simulink model "HVDCMMCInterconnection"  (R2024b)
settings: Solver=FixedStepDiscrete  StartTime=0.0  StopTime=11  RelTol=1e-3
PreLoadFcn:
  | GFLParameters_400Kv
  | HVDCMMCInterconnectionParam
StartFcn:
  | tic
StopFcn:
  | toc
values from neighbouring files (symbols this model uses):
  C_PM = 1.758e-3    (= 0.001758)    [HVDCMMCInterconnectionParam.m]
  Cfilter = 1/(Larm*wc2)    (= 4.78421193241e-05)    [HVDCMMCInterconnectionParam.m]
  Cg = 50e-9    (= 5e-08)    [HVDCMMCInterconnectionParam.m]
  Fc = Fnom*3.37    (= 168.5)    [HVDCMMCInterconnectionParam.m]
  Fnom = 50    [GFLParameters_400Kv.m]    (also in HVDCMMCInterconnectionParam.m)
  L_cable = 15e-3    (= 0.015)    [HVDCMMCInterconnectionParam.m]
  Larm = Larm_pu*(Zbase/(2*pi*Fnom))    (= 0.0529455974536)    [HVDCMMCInterconnectionParam.m]
  Limits_Qreg = [ 0.25, -0.25 ]    [HVDCMMCInterconnectionParam.m]
  Lxfo = 0.12    [HVDCMMCInterconnectionParam.m]
  Nb_PM = 36    [HVDCMMCInterconnectionParam.m]
  Pnom = 1000e6    (= 1000000000)    [HVDCMMCInterconnectionParam.m]
  Psc = Pnom*20    (= 20000000000)    [HVDCMMCInterconnectionParam.m]    (also in HVDCMMC_RunFaultAnalysis.m = gridSCLArray(k))
  R_cable = 0.5    [HVDCMMCInterconnectionParam.m]
  R_startup = 400    [HVDCMMCInterconnectionParam.m]
  Rarm = Rarm_pu*Zbase    (= 0.1663335)    [HVDCMMCInterconnectionParam.m]
  Rfilter = 1/(Cfilter*w)*30    (= 1996.002)    [HVDCMMCInterconnectionParam.m]
  Rg = 100    [HVDCMMCInterconnectionParam.m]
  Rxfo = 0.003    [HVDCMMCInterconnectionParam.m]
  Slope_Pref = 0.5    [HVDCMMCInterconnectionParam.m]
  Slope_Qref = 0.5    [HVDCMMCInterconnectionParam.m]
  Slope_Vdc_ref = Vnom_dc/5    (= 128000)    [HVDCMMCInterconnectionParam.m]
  Tbrk1_On = 0.1    [HVDCMMCInterconnectionParam.m]
  Tbrk2_On = 1.0    (= 1)    [HVDCMMCInterconnectionParam.m]
  Tdeblock = 1.5    [HVDCMMCInterconnectionParam.m]
  Tfault = 9999    [HVDCMMCInterconnectionParam.m]
  Ton_Converter2 = 4    [HVDCMMCInterconnectionParam.m]
  Ton_PQreg = 4    [HVDCMMCInterconnectionParam.m]
  Ton_VDCreg = 1.5    [HVDCMMCInterconnectionParam.m]
  Ts = Ts_Control    (= 4e-05)    [HVDCMMCInterconnectionParam.m]
  Ts_Power = 20e-6    (= 2e-05)    [HVDCMMCInterconnectionParam.m]
  Vnom_dc = 640e3    (= 640000)    [HVDCMMCInterconnectionParam.m]
  Vnom_prim = 400e3    (= 400000)    [HVDCMMCInterconnectionParam.m]
  Vnom_sec = 333e3    (= 333000)    [HVDCMMCInterconnectionParam.m]
undefined symbols (not defined in the file or in its folder): ConvCtrl, ConvPlt, DiscIntNeverNeededParam, Discrete, ee_sli_rtmsupport, Fault, gcbh, gridInverter, magnitude, Pcc, PlantSim, sps, sps_rtmsupport, spsPLL3phModel, TL, Trf
libraries: powerlib_extras x27, spsSeriesRLCBranchLib x27, simulink x14, eeGeneralControl x11, spsCurrentMeasurementLib x11, spsVoltageMeasurementLib x8, spsBreakerLib x7, eeTransforms x6, spsHalfBridgeMMCLib x6, spsSecondOrderFilterLib x4, spsabctodq0Lib x4, spsThreePhaseVIMeasurementLib x4
(part 1 of 6)
settings Model: SimulationMode=accelerator  Creator=The MathWorks, Inc.  LastModifiedBy=ke416
settings SolverCC: AlgebraicLoopSolver=TrustRegion  AutoInsertRateTranBlk=on
settings DataIOCC: SaveOutput=off  DSMLogging=off  SaveTime=off  ReturnWorkspaceOutputsName=outData
settings OptimizationCC: ReuseModelBlockBuffer=off  ExpressionDepthLimit=2147483647  LifeSpan=inf
settings DebuggingCC: CheckSSInitialOutputMsg=off  UnderspecifiedInitializationDetection=Classic  MergeDetectMultiDrivingBlocksExec=none  SolverPrmCheckMsg=warning  FcnCallInpInsideContextMsg=warning  UnconnectedInputMsg=warning  UnconnectedOutputMsg=warning  UnconnectedLineMsg=warning  AllowSymbolicDim=off  StateNameClashWarn=warning  SFUnexpectedBacktrackingDiag=warning  SFNoUnconditionalDefaultTransitionDiag=warning  SFExecutionAtInitializationDiag=none  ArithmeticOperatorsInVariantConditions=warning
settings HardwareCC: ProdBitPerPointer=32  ProdBitPerSizeT=32  ProdBitPerPtrDiffT=32  ProdLargestAtomicFloat=None  ProdIntDivRoundTo=Undefined  ProdEndianess=Unspecified  ProdWordSize=32  ProdHWDeviceType=32-bit Generic
settings ModelReferenceCC: EnableRefExpFcnMdlSchedulingChecks=on  PropagateSignalLabelsOutOfModel=off
settings SFSimCC: SimUseLocalCustomCode=off  CustomCodeUndefinedFunction=UseInterfaceOnly
settings RTWCC: RTWUseLocalCustomCode=off  GPUComputeCapability=3.5
settings CodeAppCC: StateflowObjectComments=on
settings GRTTargetCC: TargetLangStandard=C89/C90 (ANSI)  CombineOutputUpdateFcns=off  GRTInterface=on
settings ConfigComp: CovMetricSettings=dw  CovSaveCumulativeToWorkspaceVar=on  CovSaveSingleToWorkspaceVar=on  CovExternalEMLEnable=off
settings SimscapeCC: SimscapeNormalizeSystem=off

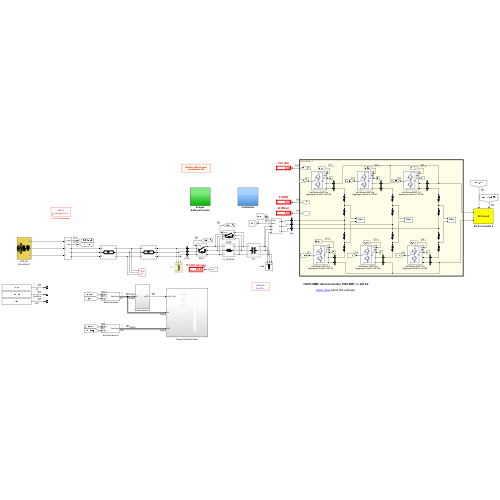
[thumbnail: Simulink's stored preview of the top-level diagram]
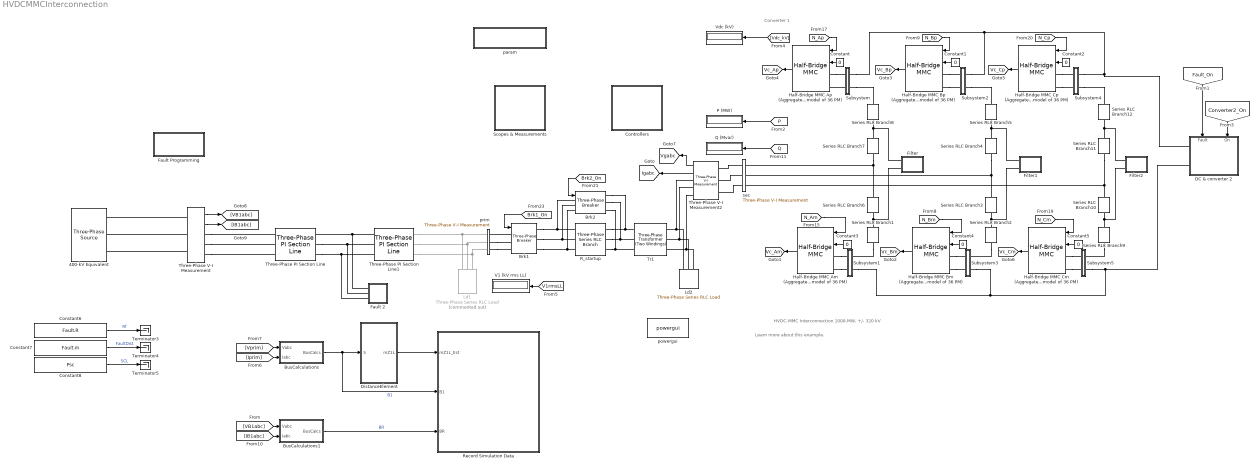
== system HVDCMMCInterconnection ==
  note: Converter 1
  note: HVDC-MMC Interconnection 1000-MW, +/- 320 kV
  note: Learn more about this example.
  400-kV Equivalent : spsThreePhaseSourceLib/Three-Phase Source  InternalConnection=Yg  VoltagePhases=off  Voltage=Vnom_prim*0.99  PhaseAngle=0  Voltage_phases=[25e3 25e3 25e3]/sqrt(3)  PhaseAngles_phases=[0 -120 +120]  Frequency=Fnom  NonIdealSource=on  SpecifyImpedance=on  Resistance=0.8929  Inductance=16.58e-3  ShortCircuitLevel=Psc  BaseVoltage=Vnom_prim  XRratio=7  BusType=swing  Pref=0  Qref=0  Prefabc=[10e3, 10e3, 10e3]  Qrefabc=[0, 0, 0]  Qmin=-inf  Qmax=inf
  Brk1 : spsThreePhaseBreakerLib/Three-Phase Breaker  InitialState=open  SwitchA=on  SwitchB=on  SwitchC=on  SwitchTimes=0.1  External=on  BreakerResistance=0.001  SnubberResistance=1e6  SnubberCapacitance=inf  Measurements=None
  Brk2 : spsThreePhaseBreakerLib/Three-Phase Breaker  InitialState=open  SwitchA=on  SwitchB=on  SwitchC=on  SwitchTimes=[30/60]*10000  External=on  BreakerResistance=0.01  SnubberResistance=1e6  SnubberCapacitance=inf  Measurements=None
  BusCalculations : Subsystem  mask{Freq=PlantSim.Freq, Ts=PlantSim.Ts}
      mask prompts: Freq "Nominal Frequency (Hz):"; Ts "Sampling Time (s):"
  BusCalculations1 : Subsystem  mask{Freq=PlantSim.Freq, Ts=PlantSim.Ts}
      mask prompts: Freq "Nominal Frequency (Hz):"; Ts "Sampling Time (s):"
  Constant{,1..5} (6 alike) : Constant  Value=0
  Constant6 : Constant  Value=Fault.R  SampleTime=-1
  Constant7 : Constant  Value=Fault.m  SampleTime=-1
  Constant8 : Constant  Value=Psc  SampleTime=-1
  Controllers : Subsystem
  DC & converter 2 : Subsystem
      settings: PortSchema="{\"entries\":[{\"content\":{\"sides\":[{\"content\":{\"connectorIds\":[\"LConn1\",\"LConn2\"]},\"type\":\"ConnectorPlacement.EquallySpacedRectSide\",\"uuid\":\"7a2c87ad-91de-4512-ad2a-35713ffc2c67\"},{\"content\":{\"connectorIds\":[],\"side\":\"RIGHT\"},\"type\":\"ConnectorPlacement.EquallySpacedRectSide\",\"uuid\":\"a4d51b8d-9b80-4f56-8990-d227af10d4d9\"},{\"content\":{\"connectorIds\":[\"In1\",\"In2\"],\"side\":\"TOP\"},\"type\":\"ConnectorPlacement.EquallySpacedRectSide\",\"uuid\":\"21e823e1-439d-404c-83ef-6279f9df48a0\"}]},\"type\":\"ConnectorPlacement.EquallySpacedConnector\",\"uuid\":\"7be36849-7bc6-4892-aa95-a5e675f45e41\"}],\"packageUris\":[\"http://schema.mathworks.com/mf0/Connector/R2020b\"],\"version\":\"1.0\"}"
      mask Display: disp('DC circuit')
  DistanceElement : Subsystem
  Fault 2 : Subsystem  mask(Fault Breaker){Ts=Ts_Power}
      mask prompts: Ts "Sample time:"
      mask Display: disp('Fault\n L1')
  Fault Programming : Subsystem  mask(Fault programming){FaultType=ABC-G, FaultLocation=L1: Protected line, ParT=[Fault.StartTime Fault.EndTime], Ts=Ts_Power}
      mask prompts: FaultType "Fault type:"; FaultLocation "Fault Location:"; ParT "Fault timing (s): [ Ton  Toff ]"; Ts "Sample time:"
      mask init:
      | switch FaultType
      | case 1
      | str='NO Fault';
      | case 2
      | str='A-G';
      | case 3
      | str='AB';
      | case 4
      | str='AB-G';
      | case 5
      | str='ABC';
      | case 6
      | str='ABC-G';
      | end
      | switch FaultLocation
      | case 1
      | str1='Protected line (L1)';
      | case 2
      | str1='Parallel line (L2)';
      | end
      | str2=sprintf('%s\n%s',str,str1);
      | Ton=ParT(1);
      | Toff=ParT(2);
      mask TypeOptions FaultType: No fault | A-G | AB | AB-G | ABC | ABC-G
      mask TypeOptions FaultLocation: L1: Protected line | L2: Parallel line
      mask Display: disp(str2)
  Filter : Subsystem
      mask Display: disp('Filter')
  Filter1 : Subsystem
      mask Display: disp('Filter')
  Filter2 : Subsystem
      mask Display: disp('Filter')
  Half-Bridge MMC Am (Aggregate model of 36 PM) : spsHalfBridgeMMCLib/Half-Bridge MMC  ModelType=Aggregate model  n=36  C=C_PM  Vc_Initial=Vc0_PM  Ron=1e-3  Rs=1e6  Cs=inf  Ron_Diode=1e-3  Rs_Diode=1e6  Cs_Diode=inf  Vf_Diode=1e-3  Rs_CurrentSource=inf  Ts=Ts_Power
  Half-Bridge MMC Ap (Aggregate model of 36 PM) : spsHalfBridgeMMCLib/Half-Bridge MMC  ModelType=Aggregate model  n=36  C=C_PM  Vc_Initial=Vc0_PM  Ron=1e-3  Rs=1e6  Cs=inf  Ron_Diode=1e-3  Rs_Diode=1e6  Cs_Diode=inf  Vf_Diode=1e-3  Rs_CurrentSource=inf  Ts=Ts_Power
  Half-Bridge MMC Bm (Aggregate model of 36 PM) : spsHalfBridgeMMCLib/Half-Bridge MMC  ModelType=Aggregate model  n=36  C=C_PM  Vc_Initial=Vc0_PM  Ron=1e-3  Rs=1e6  Cs=inf  Ron_Diode=1e-3  Rs_Diode=1e6  Cs_Diode=inf  Vf_Diode=1e-3  Rs_CurrentSource=inf  Ts=Ts_Power
  "Half-Bridge MMC Bp (Aggregate model of 36 PM) " : spsHalfBridgeMMCLib/Half-Bridge MMC  ModelType=Aggregate model  n=36  C=C_PM  Vc_Initial=Vc0_PM  Ron=1e-3  Rs=1e6  Cs=inf  Ron_Diode=1e-3  Rs_Diode=1e6  Cs_Diode=inf  Vf_Diode=1e-3  Rs_CurrentSource=inf  Ts=Ts_Power
  Half-Bridge MMC Cm (Aggregate model of 36 PM) : spsHalfBridgeMMCLib/Half-Bridge MMC  ModelType=Aggregate model  n=36  C=C_PM  Vc_Initial=Vc0_PM  Ron=1e-3  Rs=1e6  Cs=inf  Ron_Diode=1e-3  Rs_Diode=1e6  Cs_Diode=inf  Vf_Diode=1e-3  Rs_CurrentSource=inf  Ts=Ts_Power
  Half-Bridge MMC Cp (Aggregate model of 36 PM) : spsHalfBridgeMMCLib/Half-Bridge MMC  ModelType=Aggregate model  n=36  C=C_PM  Vc_Initial=Vc0_PM  Ron=1e-3  Rs=1e6  Cs=inf  Ron_Diode=1e-3  Rs_Diode=1e6  Cs_Diode=inf  Vf_Diode=1e-3  Rs_CurrentSource=inf  Ts=Ts_Power
  Ld1 : spsThreePhaseSeriesRLCLoadLib/Three-Phase Series RLC Load  Commented=on  LConnTagsString=A|B|C  Configuration=Y (grounded)  NominalVoltage=Vnom_prim  Vabc=[1e3 1e3 1e3]  Vabcp=[1e3 1e3 1e3]  NominalFrequency=Fnom  UnbalancedPower=off  ActivePower=P_Ld1  InductivePower=0  CapacitivePower=0  Pabc=[10e3 9e3 11e3]  QLabc=[100 90 110]  QCabc=[100 90 110]  Pabcp=[10e3 9e3 11e3]  QLabcp=[100 90 110]  QCabcp=[100 90 110]  Measurements=None  LoadType=constant Z
  Ld2 : spsThreePhaseSeriesRLCLoadLib/Three-Phase Series RLC Load  LConnTagsString=A|B|C  Configuration=Y (grounded)  NominalVoltage=Vnom_sec  Vabc=[1e3 1e3 1e3]  Vabcp=[1e3 1e3 1e3]  NominalFrequency=Fnom  UnbalancedPower=off  ActivePower=500e3  InductivePower=0  CapacitivePower=0  Pabc=[10e3 9e3 11e3]  QLabc=[100 90 110]  QCabc=[100 90 110]  Pabcp=[10e3 9e3 11e3]  QLabcp=[100 90 110]  QCabcp=[100 90 110]  Measurements=None  LoadType=constant Z
  P (MW) : Display
      settings: Format=bank  Decimation=5000
  Q (Mvar) : Display
      settings: Format=bank  Decimation=5000
  R_startup : spsThreePhaseSeriesRLCBranchLib/Three-Phase Series RLC Branch  LConnTagsString=A|B|C  RConnTagsString=A|B|C  BranchType=R  Resistance=R_startup  Inductance=Vnom_prim^2 / Pcc / (2*pi*Fnom)  Capacitance=1e-6  Measurements=None
  Record Simulation Data : Subsystem
  Scopes & Measurements : Subsystem
  Series RLC Branch{1..12} (12 alike) : spsSeriesRLCBranchLib/Series RLC Branch  LConnTagsString=__new0  RConnTagsString=__new0  BranchType=RL  Resistance=Rarm/2  Inductance=Larm/2  SetiL0=off  InitialCurrent=0  Capacitance=1e-6  Setx0=off  InitialVoltage=0  Measurements=None
  Subsystem : Subsystem
  Subsystem1 : Subsystem
  Subsystem2 : Subsystem
  Subsystem3 : Subsystem
  Subsystem4 : Subsystem
  Subsystem5 : Subsystem
  Terminator3 : Terminator
  Terminator4 : Terminator
  Terminator5 : Terminator
  Three-Phase PI Section Line : spsThreePhasePISectionLineLib/Three-Phase PI Section Line  LConnTagsString=a|b|c  RConnTagsString=A|B|C  Length=100*(1-Fault.m)  Frequency=Fnom  Resistances=[ 0.01273 0.3864]  Inductances="[ 0.9337e-3  4.1264e-3]"  Capacitances=[12.74e-9 7.751e-9]
  Three-Phase PI Section Line1 : spsThreePhasePISectionLineLib/Three-Phase PI Section Line  LConnTagsString=a|b|c  RConnTagsString=A|B|C  Length=100*Fault.m  Frequency=Fnom  Resistances=[ 0.01273 0.3864]  Inductances="[ 0.9337e-3  4.1264e-3]"  Capacitances=[12.74e-9 7.751e-9]
  Three-Phase V-I Measurement : spsThreePhaseVIMeasurementLib/Three-Phase V-I Measurement  VoltageMeasurement=phase-to-ground  SetLabelV=off  LabelV=Vabc  Vpu=off  VpuLL=off  CurrentMeasurement=yes  SetLabelI=off  LabelI=Iabc  Ipu=off  Pbase=100e6  Vbase=500e3  OutputType=Complex  PhasorSimulation=off  PSBequivalent=0
  Three-Phase V-I Measurement2 : spsThreePhaseVIMeasurementLib/Three-Phase V-I Measurement  VoltageMeasurement=phase-to-ground  SetLabelV=off  LabelV=Vabc  Vpu=off  VpuLL=off  CurrentMeasurement=yes  SetLabelI=off  LabelI=Iabc  Ipu=off  Pbase=100e6  Vbase=500e3  OutputType=Complex  PhasorSimulation=off  PSBequivalent=0
  Tr1 : spsThreePhaseTransformerTwoWindingsLib/Three-Phase Transformer (Two Windings)  Winding1Connection=Yg  Winding2Connection=Y  CoreType=Three single-phase transformers  SetSaturation=off  Hysteresis=off  DataFile='hysteresis'  SetInitialFlux=off  Measurements=None  UNITS=pu  NominalPower=[ Pnom , Fnom ]  Winding1="[ Vnom_prim , Rxfo/2,  Lxfo/2 ]"  Winding2="[ Vnom_sec , Rxfo/2,  Lxfo/2 ]"  Rm=1000  Lm=1000  L0=0.5  Saturation=[ 0,0 ; 0.0024,1.2 ; 1.0,1.52 ]  InitialFluxes=[ 0.8 , -0.8 , 0.7 ]  BreakLoop=off  DiscreteSolver=Trapezoidal iterative  DataType=off  TransfoNumber=1
  V1 (kV rms LL) : Display
      settings: Format=bank  Decimation=5000
  Vdc (kV) : Display
      settings: Format=bank  Decimation=5000
  param : Subsystem
      settings: OpenFcn=open('HVDCMMCInterconnectionParam')
      mask Display: disp('Double-click to open\nparameters file')
  powergui : spspowerguiLib/powergui  Priority=1  SimulationMode=Discrete  SampleTime=Ts_Power  frequency=60  Iterations=50  frequencyindice=0  Pbase=100e6  ErrMax=1e-4  UnitsV=kV  UnitsW=MW  buscounter=0  FunctionMessages=off  echomessages=off  EnableUseOfTLC=off  CurrentSourceSwitches=off  DisableSnubberDevices=off  DisableRonSwitches=off  DisableVfSwitches=off  DisplayEquations=off  AutomaticDiscreteSolvers=off  SolverType=Tustin/Backward Euler (TBE)  Interpol=off  ExternalGateDelay=off  methode=off  Ts=10  x0status=blocks  SPID=off  SwTol=0  HookPort=off  NonlinearTolerance=1e-4  nMaxIteration=100  ContinueOnMaxIteration=off  RestoreLinks=warning  ResistiveCurrentMeasurement=off  Frange=[0:2:500]  Ylog=off  Xlog=on  ShowGrid=off  save=off  variable=ZData  structure=VIprim  ZoomFFT=on  StartTime=0.15  cycles=2  DisplayStyle=1  fundamental=50  FreqAxis=on  MaxFrequency=1000  frequencyindicesteady=1  RmsSteady=1  display=off
  prim : spsThreePhaseVIMeasurementLib/Three-Phase V-I Measurement  VoltageMeasurement=phase-to-ground  SetLabelV=on  LabelV=Vprim  Vpu=off  VpuLL=off  CurrentMeasurement=yes  SetLabelI=on  LabelI=Iprim  Ipu=off  Pbase=100e6  Vbase=500e3  OutputType=Complex  PhasorSimulation=off  PSBequivalent=0
  sec : spsThreePhaseVIMeasurementLib/Three-Phase V-I Measurement  VoltageMeasurement=phase-to-ground  SetLabelV=on  LabelV=Vsec  Vpu=off  VpuLL=off  CurrentMeasurement=yes  SetLabelI=on  LabelI=Isec  Ipu=off  Pbase=100e6  Vbase=500e3  OutputType=Complex  PhasorSimulation=off  PSBequivalent=0
  tag scope: Igabc=global, Vc_Am=global, Vc_Ap=global, Vc_Bm=global, Vc_Bp=global, Vc_Cm=global, Vc_Cp=global, Vgabc=global
  wires:
  [P] -> P (MW)/1
  [N_Cp] -> Half-Bridge MMC Cp (Aggregate model of 36 PM)/1
  Half-Bridge MMC Cp (Aggregate model of 36 PM)/1 -> [Vc_Cp]
  Half-Bridge MMC Am (Aggregate model of 36 PM)/1 -> [Vc_Am]
  Half-Bridge MMC Bm (Aggregate model of 36 PM)/1 -> [Vc_Bm]
  Half-Bridge MMC Cm (Aggregate model of 36 PM)/1 -> [Vc_Cm]
  [N_Bm] -> Half-Bridge MMC Bm (Aggregate model of 36 PM)/1
  [Brk2_On] -> Brk2/1
  [Vdc_kV] -> Vdc (kV)/1
  [V1rmsLL] -> V1 (kV rms LL)/1
  [Q] -> Q (Mvar)/1
  Half-Bridge MMC Ap (Aggregate model of 36 PM)/1 -> [Vc_Ap]
  [Converter2_On] -> DC & converter 2/2(On)
  [Fault_On] -> DC & converter 2/1(Fault)
  [N_Ap] -> Half-Bridge MMC Ap (Aggregate model of 36 PM)/1
  [N_Am] -> Half-Bridge MMC Am (Aggregate model of 36 PM)/1
  "Half-Bridge MMC Bp (Aggregate model of 36 PM) "/1 -> [Vc_Bp]
  [N_Bp] -> "Half-Bridge MMC Bp (Aggregate model of 36 PM) "/1
  [N_Cm] -> Half-Bridge MMC Cm (Aggregate model of 36 PM)/1
  Constant/1 -> Half-Bridge MMC Ap (Aggregate model of 36 PM)/2
  Constant1/1 -> "Half-Bridge MMC Bp (Aggregate model of 36 PM) "/2
  Constant2/1 -> Half-Bridge MMC Cp (Aggregate model of 36 PM)/2
  Constant3/1 -> Half-Bridge MMC Am (Aggregate model of 36 PM)/2
  Constant4/1 -> Half-Bridge MMC Bm (Aggregate model of 36 PM)/2
  Constant5/1 -> Half-Bridge MMC Cm (Aggregate model of 36 PM)/2
  Three-Phase V-I Measurement2/1 -> [Vgabc]
  Three-Phase V-I Measurement2/2 -> [Igabc]
  [Brk1_On] -> Brk1/1
  BusCalculations/1(BusCalcs) -> Record Simulation Data/2(B1), DistanceElement/1(S)  "B1"
  Constant8/1 -> Terminator5/1  "SCL"
  DistanceElement/1(mZ1L) -> Record Simulation Data/1(mZ1L_Est)
  Constant7/1 -> Terminator4/1  "FaultDist"
  Constant6/1 -> Terminator3/1  "Rf"
  [Iprim] -> BusCalculations/2(Iabc)
  [Vprim] -> BusCalculations/1(Vabc)
  BusCalculations1/1(BusCalcs) -> Record Simulation Data/3(BR)  "BR"
  [VB1abc] -> BusCalculations1/1(Vabc)
  [IB1abc] -> BusCalculations1/2(Iabc)
  Three-Phase V-I Measurement/2 -> [IB1abc]
  Three-Phase V-I Measurement/1 -> [VB1abc]
  connections:
  Ld1/LConn1 -- Three-Phase PI Section Line1/RConn1 -- prim/RConn1
  Ld1/LConn2 -- Three-Phase PI Section Line1/RConn2 -- prim/RConn2
  Ld1/LConn3 -- Three-Phase PI Section Line1/RConn3 -- prim/RConn3
  Series RLC Branch7/RConn1 -- Series RLC Branch6/LConn1 -- sec/LConn1
  Series RLC Branch1/LConn1 -- Filter/LConn2 -- Series RLC Branch6/RConn1
  Series RLC Branch7/LConn1 -- Filter/LConn1 -- Series RLC Branch8/RConn1
  Half-Bridge MMC Ap (Aggregate model of 36 PM)/LConn1 -- Subsystem/LConn1
  Subsystem/LConn2 -- Half-Bridge MMC Ap (Aggregate model of 36 PM)/LConn2
  Subsystem/RConn2 -- Series RLC Branch8/LConn1
  Half-Bridge MMC Am (Aggregate model of 36 PM)/LConn2 -- Subsystem1/LConn2
  Half-Bridge MMC Am (Aggregate model of 36 PM)/LConn1 -- Subsystem1/LConn1
  Series RLC Branch1/RConn1 -- Subsystem1/RConn1
  Series RLC Branch4/RConn1 -- Series RLC Branch3/LConn1 -- sec/LConn2
  Filter1/LConn2 -- Series RLC Branch2/LConn1 -- Series RLC Branch3/RConn1
  Series RLC Branch4/LConn1 -- Filter1/LConn1 -- Series RLC Branch5/RConn1
  "Half-Bridge MMC Bp (Aggregate model of 36 PM) "/LConn2 -- Subsystem2/LConn2
  "Half-Bridge MMC Bp (Aggregate model of 36 PM) "/LConn1 -- Subsystem2/LConn1
  Subsystem2/RConn2 -- Series RLC Branch5/LConn1
  Series RLC Branch2/RConn1 -- Subsystem3/RConn1
  Half-Bridge MMC Bm (Aggregate model of 36 PM)/LConn1 -- Subsystem3/LConn1
  Half-Bridge MMC Bm (Aggregate model of 36 PM)/LConn2 -- Subsystem3/LConn2
  Series RLC Branch11/RConn1 -- Series RLC Branch10/LConn1 -- sec/LConn3
  Series RLC Branch10/RConn1 -- Filter2/LConn2 -- Series RLC Branch9/LConn1
  Series RLC Branch12/RConn1 -- Series RLC Branch11/LConn1 -- Filter2/LConn1
  Half-Bridge MMC Cp (Aggregate model of 36 PM)/LConn1 -- Subsystem4/LConn1
  Half-Bridge MMC Cm (Aggregate model of 36 PM)/LConn1 -- Subsystem5/LConn1
  Half-Bridge MMC Cm (Aggregate model of 36 PM)/LConn2 -- Subsystem5/LConn2
  Subsystem4/RConn2 -- Series RLC Branch12/LConn1
  Half-Bridge MMC Cp (Aggregate model of 36 PM)/LConn2 -- Subsystem4/LConn2
  Series RLC Branch9/RConn1 -- Subsystem5/RConn1
  Subsystem/RConn1 -- Subsystem4/RConn1 -- DC & converter 2/LConn1 -- Subsystem2/RConn1
  Subsystem1/RConn2 -- Subsystem5/RConn2 -- DC & converter 2/LConn2 -- Subsystem3/RConn2
  Ld2/LConn1 -- Three-Phase V-I Measurement2/RConn1 -- Tr1/RConn1
  Ld2/LConn2 -- Three-Phase V-I Measurement2/RConn2 -- Tr1/RConn2
  Ld2/LConn3 -- Three-Phase V-I Measurement2/RConn3 -- Tr1/RConn3
  Brk2/LConn1 -- Brk1/RConn1 -- R_startup/LConn1
  Brk2/LConn2 -- Brk1/RConn2 -- R_startup/LConn2
  Brk2/LConn3 -- Brk1/RConn3 -- R_startup/LConn3
  R_startup/RConn1 -- Brk2/RConn1 -- Tr1/LConn1
  R_startup/RConn2 -- Brk2/RConn2 -- Tr1/LConn2
  R_startup/RConn3 -- Brk2/RConn3 -- Tr1/LConn3
  Three-Phase V-I Measurement/RConn2 -- Three-Phase PI Section Line/LConn2
  Three-Phase V-I Measurement/RConn1 -- Three-Phase PI Section Line/LConn1
  Three-Phase V-I Measurement/RConn3 -- Three-Phase PI Section Line/LConn3
  Three-Phase V-I Measurement/LConn3 -- 400-kV Equivalent/RConn3
  Three-Phase V-I Measurement/LConn2 -- 400-kV Equivalent/RConn2
  Three-Phase V-I Measurement/LConn1 -- 400-kV Equivalent/RConn1
  sec/RConn1 -- Three-Phase V-I Measurement2/LConn1
  sec/RConn2 -- Three-Phase V-I Measurement2/LConn2
  sec/RConn3 -- Three-Phase V-I Measurement2/LConn3
  Brk1/LConn1 -- prim/LConn1
  prim/LConn2 -- Brk1/LConn2
  prim/LConn3 -- Brk1/LConn3
  Three-Phase PI Section Line1/LConn1 -- Fault 2/LConn1 -- Three-Phase PI Section Line/RConn1
  Three-Phase PI Section Line/RConn2 -- Fault 2/LConn2 -- Three-Phase PI Section Line1/LConn2
  Three-Phase PI Section Line/RConn3 -- Fault 2/LConn3 -- Three-Phase PI Section Line1/LConn3

== system HVDCMMCInterconnection/BusCalculations ==
  Vabc : Inport
  Iabc : Inport  Port=2
  Bus Creator : BusCreator  Inputs=6
  Bus Creator3 : BusCreator  Inputs=4
  Bus Creator4 : BusCreator  Inputs=4
  Complex2Phasor : Subsystem
  Complex2Phasor1 : Subsystem
  Demux : Demux  Outputs=3
  Demux1 : Demux  Outputs=3
  Measurement Unit (Phasor Computation) : Subsystem  mask(Measurement Unit){Ts=Ts}
      mask prompts: Ts "Sample time:"
  "Power (3ph, Instantaneous)1" : spsPower3phInstantaneousLib/Power (3ph, Instantaneous)
  SymmetricalComponentsCalc : Subsystem
  SymmetricalComponentsCalc1 : Subsystem
  BusCalcs : Outport
  wires:
  Vabc/1 -> Demux/1, Measurement Unit (Phasor Computation)/1(Vabc(t)), "Power (3ph, Instantaneous)1"/1
  Iabc/1 -> Demux1/1, Measurement Unit (Phasor Computation)/2(Iabc(t)), "Power (3ph, Instantaneous)1"/2
  "Power (3ph, Instantaneous)1"/2 -> Bus Creator/6  "Q"
  Measurement Unit (Phasor Computation)/2(" Iabc_Fund") -> SymmetricalComponentsCalc1/1(abc), Complex2Phasor1/1(complex)
  Demux1/1 -> Bus Creator4/1  "a"
  Bus Creator3/1 -> Bus Creator/1  "V"
  Demux/2 -> Bus Creator3/2  "b"
  Demux1/3 -> Bus Creator4/3  "c"
  Measurement Unit (Phasor Computation)/1(Vabc_Fund) -> Complex2Phasor/1(complex), SymmetricalComponentsCalc/1(abc)
  SymmetricalComponentsCalc1/1(ABC+-0) -> Bus Creator/4  "ISymm"
  Demux/1 -> Bus Creator3/1  "a"
  SymmetricalComponentsCalc/1(ABC+-0) -> Bus Creator/2  "VSymm"
  Bus Creator4/1 -> Bus Creator/3  "I"
  Demux1/2 -> Bus Creator4/2  "b"
  "Power (3ph, Instantaneous)1"/1 -> Bus Creator/5  "P"
  Demux/3 -> Bus Creator3/3  "c"
  Bus Creator/1 -> BusCalcs/1
  Complex2Phasor/1(Phasor) -> Bus Creator3/4  "Phasor"
  Complex2Phasor1/1(Phasor) -> Bus Creator4/4  "Phasor"

== system HVDCMMCInterconnection/BusCalculations1 ==
  Vabc : Inport
  Iabc : Inport  Port=2
  Bus Creator : BusCreator  Inputs=6
  Bus Creator3 : BusCreator  Inputs=4
  Bus Creator4 : BusCreator  Inputs=4
  Complex2Phasor : Subsystem
  Complex2Phasor1 : Subsystem
  Demux : Demux  Outputs=3
  Demux1 : Demux  Outputs=3
  Measurement Unit (Phasor Computation) : Subsystem  mask(Measurement Unit){Ts=Ts}
      mask prompts: Ts "Sample time:"
  "Power (3ph, Instantaneous)1" : spsPower3phInstantaneousLib/Power (3ph, Instantaneous)
  SymmetricalComponentsCalc : Subsystem
  SymmetricalComponentsCalc1 : Subsystem
  BusCalcs : Outport
  wires:
  Complex2Phasor1/1(Phasor) -> Bus Creator4/4  "Phasor"
  Complex2Phasor/1(Phasor) -> Bus Creator3/4  "Phasor"
  Bus Creator/1 -> BusCalcs/1
  Demux/3 -> Bus Creator3/3  "c"
  "Power (3ph, Instantaneous)1"/1 -> Bus Creator/5  "P"
  Demux1/2 -> Bus Creator4/2  "b"
  Bus Creator4/1 -> Bus Creator/3  "I"
  SymmetricalComponentsCalc/1(ABC+-0) -> Bus Creator/2  "VSymm"
  Demux/1 -> Bus Creator3/1  "a"
  SymmetricalComponentsCalc1/1(ABC+-0) -> Bus Creator/4  "ISymm"
  Measurement Unit (Phasor Computation)/1(Vabc_Fund) -> SymmetricalComponentsCalc/1(abc), Complex2Phasor/1(complex)
  Demux1/3 -> Bus Creator4/3  "c"
  Demux/2 -> Bus Creator3/2  "b"
  Bus Creator3/1 -> Bus Creator/1  "V"
  Demux1/1 -> Bus Creator4/1  "a"
  Measurement Unit (Phasor Computation)/2(" Iabc_Fund") -> Complex2Phasor1/1(complex), SymmetricalComponentsCalc1/1(abc)
  "Power (3ph, Instantaneous)1"/2 -> Bus Creator/6  "Q"
  Iabc/1 -> "Power (3ph, Instantaneous)1"/2, Measurement Unit (Phasor Computation)/2(Iabc(t)), Demux1/1
  Vabc/1 -> "Power (3ph, Instantaneous)1"/1, Measurement Unit (Phasor Computation)/1(Vabc(t)), Demux/1

== system HVDCMMCInterconnection/Controllers ==
  note: HVDC-MMC Control System
  Controllers : Subsystem  Variant=on  VariantControl=Controllers
  PWM Generators & Calculation of number of inserted modules (Nin) and number of blocked module (Nbl) : Subsystem
  Rate Transition11 : RateTransition  OutPortSampleTime=Ts_Power
  Sequencer : Subsystem
      mask Display: disp('Sequencer')
  Terminator : Terminator
  Terminator1 : Terminator
  Terminator2 : Terminator
  Unit Delay{,1..5} (6 alike) : UnitDelay  SampleTime=-1  HasFrameUpgradeWarning=on
  tag scope: N_Am=global, N_Ap=global, N_Bm=global, N_Bp=global, N_Cm=global, N_Cp=global
  wires:
  Rate Transition11/1 -> PWM Generators & Calculation of number of inserted modules (Nin) and number of blocked module (Nbl)/1(Uref_ABC)
  PWM Generators & Calculation of number of inserted modules (Nin) and number of blocked module (Nbl)/1(N_Ap) -> Unit Delay/1
  PWM Generators & Calculation of number of inserted modules (Nin) and number of blocked module (Nbl)/2(N_Bp) -> Unit Delay1/1
  PWM Generators & Calculation of number of inserted modules (Nin) and number of blocked module (Nbl)/3(N_Cp) -> Unit Delay2/1
  PWM Generators & Calculation of number of inserted modules (Nin) and number of blocked module (Nbl)/4(N_Am) -> Unit Delay3/1
  PWM Generators & Calculation of number of inserted modules (Nin) and number of blocked module (Nbl)/5(N_Bm) -> Unit Delay4/1
  PWM Generators & Calculation of number of inserted modules (Nin) and number of blocked module (Nbl)/6(N_Cm) -> Unit Delay5/1
  [Blk] -> PWM Generators & Calculation of number of inserted modules (Nin) and number of blocked module (Nbl)/2(Block)
  Unit Delay/1 -> [N_Ap]
  Unit Delay1/1 -> [N_Bp]
  Unit Delay2/1 -> [N_Cp]
  Unit Delay3/1 -> [N_Am]
  Unit Delay4/1 -> [N_Bm]
  Unit Delay5/1 -> [N_Cm]
  [Pref] -> Controllers/1(PrefPU)  "Pref"
  [Qref] -> Controllers/2(QrefPU)  "Qref"
  [Vdc1] -> Controllers/3(Vdc)
  [Vgabc] -> Controllers/4(Vsec)
  [Igabc] -> Controllers/5(Isec)
  [Vprim] -> Controllers/6(VPcc)
  Controllers/1(Uref) -> Rate Transition11/1  "Uref_GFL"
  Controllers/2(Pmeas) -> Terminator/1
  Controllers/3(Qmeas) -> Terminator1/1
  Controllers/4(fmeas) -> Terminator2/1

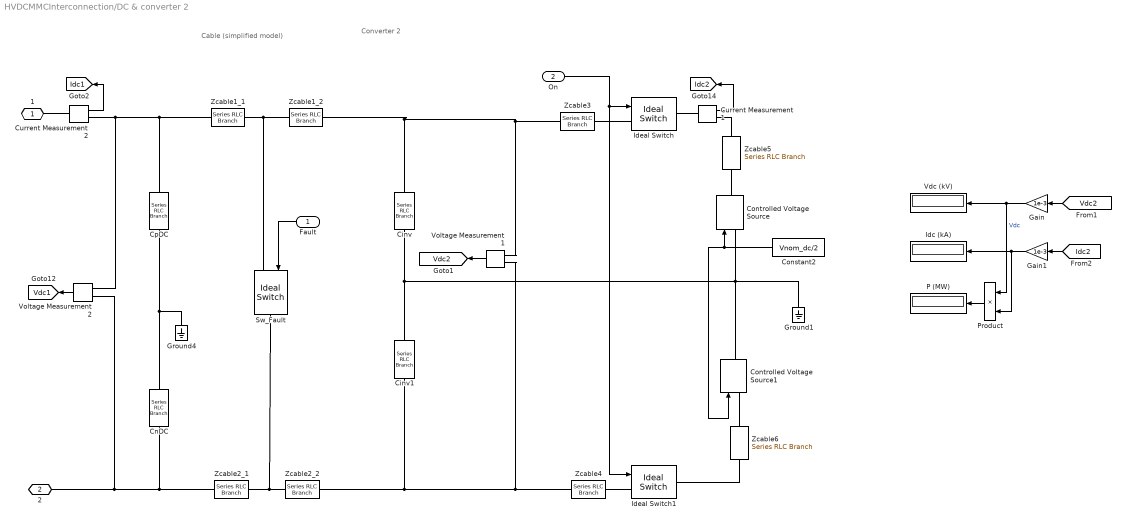
== system HVDCMMCInterconnection/DC & converter 2 ==
  note: Cable (simplified model)
  note: Converter 2
  Fault : Inport
  On : Inport  Port=2
  Cinv : spsSeriesRLCBranchLib/Series RLC Branch  LConnTagsString=__new0  RConnTagsString=__new0  BranchType=RC  Resistance=1e-3  Inductance=1e-3  SetiL0=off  InitialCurrent=0  Capacitance=C_PM/Nb_PM*3  Setx0=off  InitialVoltage=Vnom_dc/2  Measurements=None
  Cinv1 : spsSeriesRLCBranchLib/Series RLC Branch  LConnTagsString=__new0  RConnTagsString=__new0  BranchType=RC  Resistance=1e-3  Inductance=1e-3  SetiL0=off  InitialCurrent=0  Capacitance=C_PM/Nb_PM*3  Setx0=off  InitialVoltage=Vnom_dc/2  Measurements=None
  CnDC : spsSeriesRLCBranchLib/Series RLC Branch  LConnTagsString=__new0  RConnTagsString=__new0  BranchType=RC  Resistance=Rg  Inductance=1e-3  SetiL0=off  InitialCurrent=0  Capacitance=Cg  Setx0=off  InitialVoltage=Vnom_dc/2  Measurements=None
  Constant2 : Constant  Value=Vnom_dc/2  SampleTime=Ts_Power
  Controlled Voltage Source : spsControlledVoltageSourceLib/Controlled Voltage Source  Initialize=off  Source_Type=AC  Amplitude=0  Phase=0  Frequency=0  Measurements=None
  Controlled Voltage Source1 : spsControlledVoltageSourceLib/Controlled Voltage Source  Initialize=off  Source_Type=AC  Amplitude=0  Phase=0  Frequency=0  Measurements=None
  CpDC : spsSeriesRLCBranchLib/Series RLC Branch  LConnTagsString=__new0  RConnTagsString=__new0  BranchType=RC  Resistance=Rg  Inductance=1e-3  SetiL0=off  InitialCurrent=0  Capacitance=Cg  Setx0=off  InitialVoltage=Vnom_dc/2  Measurements=None
  Current Measurement1 : spsCurrentMeasurementLib/Current Measurement  PhasorSimulation=off  OutputType=Complex  PSBequivalent=0
  Current Measurement2 : spsCurrentMeasurementLib/Current Measurement  PhasorSimulation=off  OutputType=Complex  PSBequivalent=0
  Gain : Gain  Gain=1e-3
  Gain1 : Gain  Gain=1e-3
  Ground1 : spsGroundLib/Ground  LConnTagsString=a
  Ground4 : spsGroundLib/Ground  LConnTagsString=a
  Idc (kA) : Display
      settings: Format=bank  Decimation=5000
  Ideal Switch : spsIdealSwitchLib/Ideal Switch  Ron=0.001  Lon=0  IC=0  Rs=1e6  Cs=inf  Measurements=off
  Ideal Switch1 : spsIdealSwitchLib/Ideal Switch  Ron=0.001  Lon=0  IC=0  Rs=1e6  Cs=inf  Measurements=off
  P (MW) : Display
      settings: Format=bank  Decimation=5000
  Product : Product
  Sw_Fault : spsIdealSwitchLib/Ideal Switch  Ron=Rfault  Lon=0  IC=0  Rs=1e6  Cs=inf  Measurements=off
  Vdc (kV) : Display
      settings: Format=bank  Decimation=5000
  Voltage Measurement1 : spsVoltageMeasurementLib/Voltage Measurement  PhasorSimulation=off  OutputType=Complex  PSBequivalent=0
  Voltage Measurement2 : spsVoltageMeasurementLib/Voltage Measurement  PhasorSimulation=off  OutputType=Complex  PSBequivalent=0
  Zcable1_1 : spsSeriesRLCBranchLib/Series RLC Branch  LConnTagsString=__new0  RConnTagsString=__new0  BranchType=RL  Resistance=R_cable/2  Inductance=L_cable/2  SetiL0=off  InitialCurrent=0  Capacitance=1e-6  Setx0=off  InitialVoltage=0  Measurements=None
  Zcable1_2 : spsSeriesRLCBranchLib/Series RLC Branch  LConnTagsString=__new0  RConnTagsString=__new0  BranchType=RL  Resistance=R_cable/2  Inductance=L_cable/2  SetiL0=off  InitialCurrent=0  Capacitance=1e-6  Setx0=off  InitialVoltage=0  Measurements=None
  Zcable2_1 : spsSeriesRLCBranchLib/Series RLC Branch  LConnTagsString=__new0  RConnTagsString=__new0  BranchType=RL  Resistance=R_cable/2  Inductance=L_cable/2  SetiL0=off  InitialCurrent=0  Capacitance=1e-6  Setx0=off  InitialVoltage=0  Measurements=None
  Zcable2_2 : spsSeriesRLCBranchLib/Series RLC Branch  LConnTagsString=__new0  RConnTagsString=__new0  BranchType=RL  Resistance=R_cable/2  Inductance=L_cable/2  SetiL0=off  InitialCurrent=0  Capacitance=1e-6  Setx0=off  InitialVoltage=0  Measurements=None
  Zcable3 : spsSeriesRLCBranchLib/Series RLC Branch  LConnTagsString=__new0  RConnTagsString=__new0  BranchType=R  Resistance=1e-3  Inductance=1e-3  SetiL0=off  InitialCurrent=0  Capacitance=1e-6  Setx0=off  InitialVoltage=0  Measurements=None
  Zcable4 : spsSeriesRLCBranchLib/Series RLC Branch  LConnTagsString=__new0  RConnTagsString=__new0  BranchType=R  Resistance=1e-3  Inductance=1e-3  SetiL0=off  InitialCurrent=0  Capacitance=1e-6  Setx0=off  InitialVoltage=0  Measurements=None
  Zcable5 : spsSeriesRLCBranchLib/Series RLC Branch  LConnTagsString=__new0  RConnTagsString=__new0  BranchType=RL  Resistance=1e-2  Inductance=1e-4  SetiL0=off  InitialCurrent=0  Capacitance=1e-6  Setx0=off  InitialVoltage=0  Measurements=None
  Zcable6 : spsSeriesRLCBranchLib/Series RLC Branch  LConnTagsString=__new0  RConnTagsString=__new0  BranchType=RL  Resistance=1e-2  Inductance=1e-4  SetiL0=off  InitialCurrent=0  Capacitance=1e-6  Setx0=off  InitialVoltage=0  Measurements=None
  1 : PMIOPort  Side=Left
  2 : PMIOPort  Port=2  Side=Left
  tag scope: Idc1=global, Idc2=global, Vdc1=global, Vdc2=global
  wires:
  Voltage Measurement2/1 -> [Vdc1]
  Constant2/1 -> Controlled Voltage Source1/1, Controlled Voltage Source/1
  Voltage Measurement1/1 -> [Vdc2]
  Gain/1 -> Product/1, Vdc (kV)/1  "Vdc"
  Gain1/1 -> Product/2, Idc (kA)/1
  [Vdc2] -> Gain/1
  [Idc2] -> Gain1/1
  Product/1 -> P (MW)/1
  Current Measurement1/1 -> [Idc2]
  Current Measurement2/1 -> [Idc1]
  On/1 -> Ideal Switch1/1, Ideal Switch/1
  Fault/1 -> Sw_Fault/1
  connections:
  Voltage Measurement1/LConn1 -- Zcable1_2/LConn1 -- Cinv/LConn1 -- Zcable3/RConn1
  Controlled Voltage Source1/RConn1 -- Ground1/LConn1 -- Cinv1/LConn1 -- Cinv/RConn1 -- Controlled Voltage Source/LConn1
  Ground4/LConn1 -- CnDC/LConn1 -- CpDC/RConn1
  Zcable2_1/RConn1 -- CnDC/RConn1 -- Voltage Measurement2/LConn2 -- 2/RConn1
  Zcable2_2/RConn1 -- Sw_Fault/RConn1 -- Zcable2_1/LConn1
  Ideal Switch/LConn1 -- Zcable3/LConn1
  Ideal Switch1/LConn1 -- Zcable4/LConn1
  Zcable1_1/RConn1 -- Voltage Measurement2/LConn1 -- Current Measurement2/RConn1 -- CpDC/LConn1
  Ideal Switch/RConn1 -- Current Measurement1/LConn1
  Zcable5/LConn1 -- Current Measurement1/RConn1
  Zcable5/RConn1 -- Controlled Voltage Source/RConn1
  Zcable6/LConn1 -- Controlled Voltage Source1/LConn1
  Zcable6/RConn1 -- Ideal Switch1/RConn1
  1/RConn1 -- Current Measurement2/LConn1
  Zcable1_1/LConn1 -- Zcable1_2/RConn1 -- Sw_Fault/LConn1
  Zcable2_2/LConn1 -- Cinv1/RConn1 -- Zcable4/RConn1 -- Voltage Measurement1/LConn2

== system HVDCMMCInterconnection/DistanceElement ==
  S : Inport
  Abs : Abs  SaturateOnIntegerOverflow=off
  Add : Sum
  Bus Selector : BusSelector  OutputSignals=V.Phasor.a.mag,V.Phasor.a.phase,I.Phasor.a.mag,I.Phasor.a.phase,ISymm.A.mag.zero,ISymm.A.phase.zero
  Constant : Constant  Value=1+eps*1i  SampleTime=-1
  Divide : Product  Inputs=*/
  Gain : Gain  Gain=TL.K0
  Gain2 : Gain  Gain=pi/180
  Gain3 : Gain  Gain=pi/180
  Gain4 : Gain  Gain=pi/180
  Magnitude-Angle to Complex : MagnitudeAngleToComplex
  Magnitude-Angle to Complex1 : MagnitudeAngleToComplex
  Magnitude-Angle to Complex2 : MagnitudeAngleToComplex
  Switch : Switch  Criteria=u2 ~= 0  SaturateOnIntegerOverflow=off  InputSameDT=off
  mZ1L : Outport
  wires:
  Magnitude-Angle to Complex1/1 -> Add/1  "IaS"
  Bus Selector/1 -> Magnitude-Angle to Complex/1  "<mag>"
  Divide/1 -> mZ1L/1  "mZ1L_Est"
  Add/1 -> Abs/1, Switch/1  "IaS+I0SK0"
  Bus Selector/3 -> Magnitude-Angle to Complex1/1  "<mag>"
  Bus Selector/2 -> Gain2/1  "<phase>"
  Magnitude-Angle to Complex2/1 -> Gain/1  "I0S"
  Magnitude-Angle to Complex/1 -> Divide/1  "VaS"
  Gain/1 -> Add/2
  Bus Selector/4 -> Gain3/1  "<phase>"
  Bus Selector/6 -> Gain4/1  "<zero>"
  Bus Selector/5 -> Magnitude-Angle to Complex2/1  "<zero>"
  S/1 -> Bus Selector/1
  Gain2/1 -> Magnitude-Angle to Complex/2
  Gain3/1 -> Magnitude-Angle to Complex1/2
  Gain4/1 -> Magnitude-Angle to Complex2/2
  Constant/1 -> Switch/3
  Switch/1 -> Divide/2
  Abs/1 -> Switch/2

== system HVDCMMCInterconnection/Fault 2 ==
  BreakerA : spsBreakerLib/Breaker  InitialState=0  SwitchingTimes="[ 4/60  5/60 ]"  External=on  BreakerResistance=0.001  SnubberResistance=1e6  SnubberCapacitance=inf  Measurements=None  MoreParameters=off  NoBreakLoop=off
      settings: AttributesFormatString=\n
  BreakerB : spsBreakerLib/Breaker  InitialState=0  SwitchingTimes="[ 4/60  5/60 ]"  External=on  BreakerResistance=0.001  SnubberResistance=1e6  SnubberCapacitance=inf  Measurements=None  MoreParameters=off  NoBreakLoop=off
      settings: AttributesFormatString=\n
  BreakerC : spsBreakerLib/Breaker  InitialState=0  SwitchingTimes="[ 4/60  5/60 ]"  External=on  BreakerResistance=0.001  SnubberResistance=1e6  SnubberCapacitance=inf  Measurements=None  MoreParameters=off  NoBreakLoop=off
      settings: AttributesFormatString=\n
  BreakerN : spsBreakerLib/Breaker  InitialState=0  SwitchingTimes="[ 4/60  5/60 ]"  External=on  BreakerResistance=0.001  SnubberResistance=1e6  SnubberCapacitance=inf  Measurements=None  MoreParameters=off  NoBreakLoop=off
      settings: AttributesFormatString=\n
  Demux : Demux
      settings: DisplayOption=none
  Ground : spsGroundLib/Ground  LConnTagsString=a  RConnTagsString=__newr0
  Series RLC Branch : spsSeriesRLCBranchLib/Series RLC Branch  LConnTagsString=__new0  RConnTagsString=__new0  BranchType=R  Resistance=Fault.R  Inductance=1e-3  SetiL0=off  InitialCurrent=0  Capacitance=1e-6  Setx0=off  InitialVoltage=0  Measurements=None
  Series RLC Branch1 : spsSeriesRLCBranchLib/Series RLC Branch  LConnTagsString=__new0  RConnTagsString=__new0  BranchType=R  Resistance=Fault.R  Inductance=1e-3  SetiL0=off  InitialCurrent=0  Capacitance=1e-6  Setx0=off  InitialVoltage=0  Measurements=None
  Series RLC Branch2 : spsSeriesRLCBranchLib/Series RLC Branch  LConnTagsString=__new0  RConnTagsString=__new0  BranchType=R  Resistance=Fault.R  Inductance=1e-3  SetiL0=off  InitialCurrent=0  Capacitance=1e-6  Setx0=off  InitialVoltage=0  Measurements=None
  A : PMIOPort  Side=Left
  B : PMIOPort  Port=2  Side=Left
  C : PMIOPort  Port=3  Side=Left
  wires:
  [Fault_L1] -> Demux/1
  Demux/4 -> BreakerN/1
  Demux/3 -> BreakerC/1
  Demux/2 -> BreakerB/1
  Demux/1 -> BreakerA/1
  connections:
  BreakerN/RConn1 -- Ground/LConn1
  C/RConn1 -- BreakerC/LConn1
  B/RConn1 -- BreakerB/LConn1
  A/RConn1 -- BreakerA/LConn1
  BreakerN/LConn1 -- Series RLC Branch1/RConn1 -- Series RLC Branch2/RConn1 -- Series RLC Branch/RConn1
  Series RLC Branch/LConn1 -- BreakerA/RConn1
  Series RLC Branch1/LConn1 -- BreakerB/RConn1
  BreakerC/RConn1 -- Series RLC Branch2/LConn1

== system HVDCMMCInterconnection/Fault Programming ==
  Constant : Constant  Value=[1 0 0 1]
  Constant1 : Constant  Value=[1 1 0 0]
  Constant10 : Constant  Value=[0 0 0 0]
  Constant2 : Constant  Value=[1 1 0 1]
  Constant3 : Constant  Value=[1 1 1 0]
  Constant4 : Constant  Value=[1 1 1 1]
  Constant5 : Constant  Value=FaultType
  Constant6 : Constant  Value=FaultLocation
  Constant7 : Constant  Value=[1 0]  OutDataTypeStr=boolean
  Constant8 : Constant  Value=[0 1]  OutDataTypeStr=boolean
  Data Type Conversion : DataTypeConversion  SaturateOnIntegerOverflow=off  RndMeth=Floor
  Demux : Demux  Outputs=2
      settings: DisplayOption=none
  Logical Operator : Logic
  Logical Operator1 : Logic
  Multiport Switch : MultiPortSwitch  Inputs=6
  Multiport Switch1 : MultiPortSwitch  Inputs=2
  Product : Product  InputSameDT=on  SaturateOnIntegerOverflow=on  OutDataTypeStr=Inherit: Same as first input
  Step_Off : Step  Time=Toff  After=-1  SampleTime=0
  Step_On : Step  Time=Ton  SampleTime=Ts
  Sum : Sum  Inputs=|++  InputSameDT=on  SaturateOnIntegerOverflow=on  OutDataTypeStr=Inherit: Same as first input
  tag scope: Fault_L1=global, Fault_L2=global, Fault_Signal=global
  wires:
  Constant10/1 -> Multiport Switch/2
  Constant/1 -> Multiport Switch/3
  Constant1/1 -> Multiport Switch/4
  Constant2/1 -> Multiport Switch/5
  Constant3/1 -> Multiport Switch/6
  Constant4/1 -> Multiport Switch/7
  Demux/2 -> Logical Operator1/2
  Demux/1 -> Logical Operator/2
  Constant8/1 -> Multiport Switch1/3
  Constant7/1 -> Multiport Switch1/2
  Multiport Switch1/1 -> Demux/1
  Product/1 -> Data Type Conversion/1
  Logical Operator1/1 -> [Fault_L2]
  Logical Operator/1 -> [Fault_L1]
  Constant6/1 -> Multiport Switch1/1
  Constant5/1 -> Multiport Switch/1
  Multiport Switch/1 -> Product/2
  Sum/1 -> [Fault_Signal], Product/1
  Step_Off/1 -> Sum/2
  Step_On/1 -> Sum/1
  Data Type Conversion/1 -> Logical Operator/1, Logical Operator1/1

== system HVDCMMCInterconnection/Filter ==
  Breaker : spsBreakerLib/Breaker  InitialState=1  SwitchingTimes=Topen_Filter  External=off  BreakerResistance=0.001  SnubberResistance=1e6  SnubberCapacitance=inf  Measurements=None  MoreParameters=on  NoBreakLoop=off
  Current Measurement6 : spsCurrentMeasurementLib/Current Measurement  PhasorSimulation=off  OutputType=Complex  PSBequivalent=0
  Parallel RLC Branch : spsParallelRLCBranchLib/Parallel RLC Branch  LConnTagsString=a  RConnTagsString=__new0  BranchType=RC  Resistance=Rfilter  Inductance=1e-3  SetiL0=off  InitialCurrent=0  Capacitance=Cfilter  Setx0=off  InitialVoltage=0  Measurements=None
  1 : PMIOPort  Side=Left
  2 : PMIOPort  Port=2  Side=Left
  tag scope: Ifilter_A=global
  wires:
  Current Measurement6/1 -> [Ifilter_A]
  connections:
  Parallel RLC Branch/RConn1 -- 2/RConn1
  Current Measurement6/RConn1 -- Parallel RLC Branch/LConn1
  1/RConn1 -- Breaker/LConn1
  Breaker/RConn1 -- Current Measurement6/LConn1

== system HVDCMMCInterconnection/Filter1 ==
  Breaker : spsBreakerLib/Breaker  InitialState=1  SwitchingTimes=Topen_Filter  External=off  BreakerResistance=0.001  SnubberResistance=1e6  SnubberCapacitance=inf  Measurements=None  MoreParameters=on  NoBreakLoop=off
  Current Measurement6 : spsCurrentMeasurementLib/Current Measurement  PhasorSimulation=off  OutputType=Complex  PSBequivalent=0
  Parallel RLC Branch : spsParallelRLCBranchLib/Parallel RLC Branch  LConnTagsString=a  RConnTagsString=__new0  BranchType=RC  Resistance=Rfilter  Inductance=1e-3  SetiL0=off  InitialCurrent=0  Capacitance=Cfilter  Setx0=off  InitialVoltage=0  Measurements=None
  1 : PMIOPort  Side=Left
  2 : PMIOPort  Port=2  Side=Left
  tag scope: Ifilter_B=global
  wires:
  Current Measurement6/1 -> [Ifilter_B]
  connections:
  Current Measurement6/RConn1 -- Parallel RLC Branch/LConn1
  Parallel RLC Branch/RConn1 -- 2/RConn1
  1/RConn1 -- Breaker/LConn1
  Breaker/RConn1 -- Current Measurement6/LConn1

== system HVDCMMCInterconnection/Filter2 ==
  Breaker : spsBreakerLib/Breaker  InitialState=1  SwitchingTimes=Topen_Filter  External=off  BreakerResistance=0.001  SnubberResistance=1e6  SnubberCapacitance=inf  Measurements=None  MoreParameters=on  NoBreakLoop=off
  Current Measurement6 : spsCurrentMeasurementLib/Current Measurement  PhasorSimulation=off  OutputType=Complex  PSBequivalent=0
  Parallel RLC Branch : spsParallelRLCBranchLib/Parallel RLC Branch  LConnTagsString=a  RConnTagsString=__new0  BranchType=RC  Resistance=Rfilter  Inductance=1e-3  SetiL0=off  InitialCurrent=0  Capacitance=Cfilter  Setx0=off  InitialVoltage=0  Measurements=None
  1 : PMIOPort  Side=Left
  2 : PMIOPort  Port=2  Side=Left
  tag scope: Ifilter_C=global
  wires:
  Current Measurement6/1 -> [Ifilter_C]
  connections:
  Parallel RLC Branch/RConn1 -- 2/RConn1
  Current Measurement6/RConn1 -- Parallel RLC Branch/LConn1
  Current Measurement6/LConn1 -- Breaker/RConn1
  1/RConn1 -- Breaker/LConn1

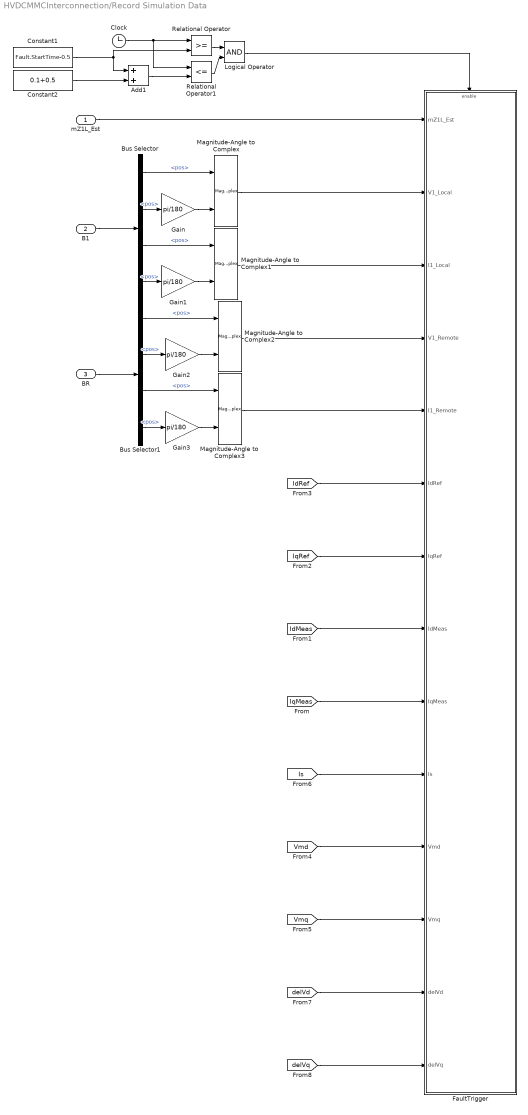
== system HVDCMMCInterconnection/Record Simulation Data ==
  mZ1L_Est : Inport
  B1 : Inport  Port=2
  BR : Inport  Port=3
  Add1 : Sum
  Bus Selector : BusSelector  OutputSignals=VSymm.A.mag.pos,VSymm.A.phase.pos,ISymm.A.mag.pos,ISymm.A.phase.pos
  Bus Selector1 : BusSelector  OutputSignals=VSymm.A.mag.pos,VSymm.A.phase.pos,ISymm.A.mag.pos,ISymm.A.phase.pos
  Clock : Clock
  Constant1 : Constant  Value=Fault.StartTime-0.5  SampleTime=-1
  Constant2 : Constant  Value=0.1+0.5  SampleTime=-1
  FaultTrigger : Subsystem
  Gain{,1..3} (4 alike) : Gain  Gain=pi/180
  Logical Operator : Logic  AllPortsSameDT=off  OutDataTypeStr=boolean
  Magnitude-Angle to Complex{,1..3} (4 alike) : MagnitudeAngleToComplex
  Relational Operator : RelationalOperator  OutDataTypeStr=boolean  RndMeth=Simplest  InputSameDT=off
  Relational Operator1 : RelationalOperator  Operator=<=  OutDataTypeStr=boolean  RndMeth=Simplest  InputSameDT=off
  wires:
  Relational Operator/1 -> Logical Operator/1
  Constant1/1 -> Add1/1, Relational Operator/2
  Relational Operator1/1 -> Logical Operator/2
  Add1/1 -> Relational Operator1/2
  Constant2/1 -> Add1/2
  Logical Operator/1 -> FaultTrigger/Enable
  Clock/1 -> Relational Operator1/1, Relational Operator/1
  mZ1L_Est/1 -> FaultTrigger/1(mZ1L_Est)
  B1/1 -> Bus Selector/1
  BR/1 -> Bus Selector1/1
  Bus Selector/2 -> Gain/1  "<pos>"
  Bus Selector/1 -> Magnitude-Angle to Complex/1  "<pos>"
  Gain/1 -> Magnitude-Angle to Complex/2
  Gain1/1 -> Magnitude-Angle to Complex1/2
  Bus Selector/3 -> Magnitude-Angle to Complex1/1  "<pos>"
  Bus Selector/4 -> Gain1/1  "<pos>"
  Bus Selector1/3 -> Magnitude-Angle to Complex3/1  "<pos>"
  Gain3/1 -> Magnitude-Angle to Complex3/2
  Gain2/1 -> Magnitude-Angle to Complex2/2
  Bus Selector1/2 -> Gain2/1  "<pos>"
  Bus Selector1/1 -> Magnitude-Angle to Complex2/1  "<pos>"
  Bus Selector1/4 -> Gain3/1  "<pos>"
  Magnitude-Angle to Complex/1 -> FaultTrigger/2(V1_Local)
  Magnitude-Angle to Complex1/1 -> FaultTrigger/3(I1_Local)
  Magnitude-Angle to Complex2/1 -> FaultTrigger/4(V1_Remote)
  Magnitude-Angle to Complex3/1 -> FaultTrigger/5(I1_Remote)
  [IdRef] -> FaultTrigger/6(IdRef)
  [IqRef] -> FaultTrigger/7(IqRef)
  [IdMeas] -> FaultTrigger/8(IdMeas)
  [IqMeas] -> FaultTrigger/9(IqMeas)
  [Is] -> FaultTrigger/10(Is)
  [Vmd] -> FaultTrigger/11(Vmd)
  [Vmq] -> FaultTrigger/12(Vmq)
  [delVd] -> FaultTrigger/13(delVd)
  [delVq] -> FaultTrigger/14(delVq)

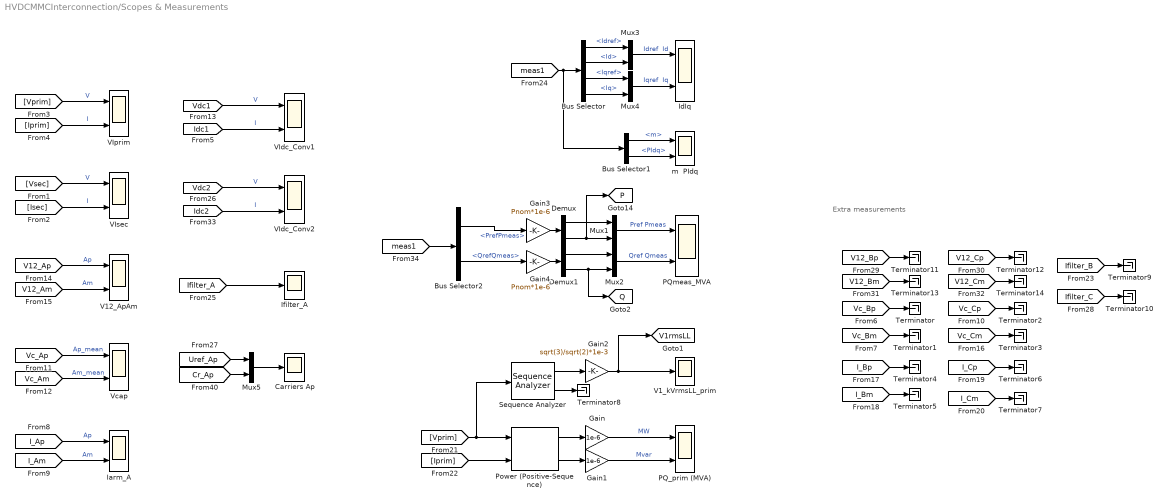
== system HVDCMMCInterconnection/Scopes & Measurements ==
  note: Extra measurements
  Bus Selector : BusSelector  OutputSignals=Idref,Id,Iqref,Iq
  Bus Selector1 : BusSelector  OutputSignals=m,PIdq
  Bus Selector2 : BusSelector  OutputSignals=PrefPmeas,QrefQmeas
  Carriers Ap : Scope
  Demux : Demux  Outputs=2
  Demux1 : Demux  Outputs=2
  Gain : Gain  Gain=1e-6
  Gain1 : Gain  Gain=1e-6
  Gain2 : Gain  Gain=sqrt(3)/sqrt(2)*1e-3
  Gain3 : Gain  Gain=Pnom*1e-6
  Gain4 : Gain  Gain=Pnom*1e-6
  Iarm_A : Scope  NumInputPorts=2
  IdIq : Scope  NumInputPorts=2
  Ifilter_A : Scope
  Mux{1..5} (5 alike) : Mux  Inputs=2
  PQ_prim (MVA) : Scope  NumInputPorts=2
  PQmeas_MVA : Scope  NumInputPorts=2
  Power (Positive-Sequence) : spsPowerPositiveSequenceLib/Power (Positive-Sequence)  Freq=Fnom  Vinit=[0, 0]  Iinit=[0, 0]  Ts=Ts_Power
  Sequence Analyzer : spsSequenceAnalyzerLib/Sequence Analyzer  Freq=Fnom  n=1  seq=Positive  InInit=[1, 0]  Ts=Ts_Power
  Terminator{,1..14} (15 alike) : Terminator
  V12_ApAm : Scope  NumInputPorts=2
  V1_kVrmsLL_prim : Scope
  VIdc_Conv1 : Scope  NumInputPorts=2
  VIdc_Conv2 : Scope  NumInputPorts=2
  VIprim : Scope  NumInputPorts=2
  VIsec : Scope  NumInputPorts=2
  Vcap : Scope  NumInputPorts=2
  m  PIdq : Scope  NumInputPorts=2
  tag scope: P=global, Q=global, V1rmsLL=global
  wires:
  Mux5/1 -> Carriers Ap/1
  [Cr_Ap] -> Mux5/2
  [Uref_Ap] -> Mux5/1
  [Vc_Am] -> Vcap/2  "Am_mean"
  [Vc_Ap] -> Vcap/1  "Ap_mean"
  [Idc2] -> VIdc_Conv2/2  "I"
  [Vdc2] -> VIdc_Conv2/1  "V"
  Gain4/1 -> Demux1/1
  Gain3/1 -> Demux/1
  Mux2/1 -> PQmeas_MVA/2  "Qref Qmeas"
  Bus Selector2/2 -> Gain4/1  "<QrefQmeas>"
  Bus Selector2/1 -> Gain3/1  "<PrefPmeas>"
  Mux1/1 -> PQmeas_MVA/1  "Pref Pmeas"
  [meas1] -> Bus Selector2/1
  Gain2/1 -> V1_kVrmsLL_prim/1, [V1rmsLL]
  Gain1/1 -> PQ_prim (MVA)/2  "Mvar"
  Gain/1 -> PQ_prim (MVA)/1  "MW"
  [V12_Cm] -> Terminator14/1
  [V12_Bm] -> Terminator13/1
  [V12_Cp] -> Terminator12/1
  [V12_Bp] -> Terminator11/1
  [Ifilter_C] -> Terminator10/1
  [Ifilter_B] -> Terminator9/1
  Sequence Analyzer/1 -> Gain2/1
  Power (Positive-Sequence)/2 -> Gain1/1
  Power (Positive-Sequence)/1 -> Gain/1
  Sequence Analyzer/2 -> Terminator8/1
  [Iprim] -> Power (Positive-Sequence)/2
  [Vprim] -> Power (Positive-Sequence)/1, Sequence Analyzer/1
  [Idc1] -> VIdc_Conv1/2  "I"
  [Vdc1] -> VIdc_Conv1/1  "V"
  [Ifilter_A] -> Ifilter_A/1
  Bus Selector/4 -> Mux4/2  "<Iq>"
  Bus Selector/3 -> Mux4/1  "<Iqref>"
  Bus Selector/2 -> Mux3/2  "<Id>"
  Bus Selector/1 -> Mux3/1  "<Idref>"
  Mux4/1 -> IdIq/2  "Iqref  Iq"
  Mux3/1 -> IdIq/1  "Idref  Id"
  Bus Selector1/2 -> m  PIdq/2  "<PIdq>"
  Bus Selector1/1 -> m  PIdq/1  "<m>"
  [meas1] -> Bus Selector/1, Bus Selector1/1
  [I_Cm] -> Terminator7/1
  [I_Cp] -> Terminator6/1
  [I_Bm] -> Terminator5/1
  [I_Bp] -> Terminator4/1
  [I_Am] -> Iarm_A/2  "Am"
  [I_Ap] -> Iarm_A/1  "Ap"
  [Vc_Cm] -> Terminator3/1
  [Vc_Cp] -> Terminator2/1
  [Vc_Bm] -> Terminator1/1
  [Vc_Bp] -> Terminator/1
  [V12_Am] -> V12_ApAm/2  "Am"
  [V12_Ap] -> V12_ApAm/1  "Ap"
  [Vsec] -> VIsec/1  "V"
  [Isec] -> VIsec/2  "I"
  [Vprim] -> VIprim/1  "V"
  [Iprim] -> VIprim/2  "I"
  Demux/1 -> Mux1/1
  Demux/2 -> [P], Mux1/2
  Demux1/1 -> Mux2/1
  Demux1/2 -> [Q], Mux2/2

== system HVDCMMCInterconnection/Subsystem ==
  Current Measurement1 : spsCurrentMeasurementLib/Current Measurement  PhasorSimulation=off  OutputType=Complex  PSBequivalent=0
  Voltage Measurement : spsVoltageMeasurementLib/Voltage Measurement  PhasorSimulation=off  OutputType=Complex  PSBequivalent=0
  I1 : PMIOPort  Side=Left
  I2 : PMIOPort  Port=2  Side=Left
  O1 : PMIOPort  Port=3  Side=Right
  O2 : PMIOPort  Port=4  Side=Right
  tag scope: I_Ap=global, V12_Ap=global
  wires:
  Current Measurement1/1 -> [I_Ap]
  Voltage Measurement/1 -> [V12_Ap]
  connections:
  Current Measurement1/RConn1 -- Voltage Measurement/LConn1 -- I1/RConn1
  Current Measurement1/LConn1 -- O1/RConn1
  I2/RConn1 -- Voltage Measurement/LConn2 -- O2/RConn1

== system HVDCMMCInterconnection/Subsystem1 ==
  Current Measurement1 : spsCurrentMeasurementLib/Current Measurement  PhasorSimulation=off  OutputType=Complex  PSBequivalent=0
  Voltage Measurement : spsVoltageMeasurementLib/Voltage Measurement  PhasorSimulation=off  OutputType=Complex  PSBequivalent=0
  I1 : PMIOPort  Side=Left
  I2 : PMIOPort  Port=2  Side=Left
  O1 : PMIOPort  Port=3  Side=Right
  O2 : PMIOPort  Port=4  Side=Right
  tag scope: I_Am=global, V12_Am=global
  wires:
  Voltage Measurement/1 -> [V12_Am]
  Current Measurement1/1 -> [I_Am]
  connections:
  Voltage Measurement/LConn2 -- O2/RConn1 -- I2/RConn1
  Current Measurement1/LConn1 -- O1/RConn1
  Voltage Measurement/LConn1 -- Current Measurement1/RConn1 -- I1/RConn1
